simulink model "vanderpol"  (R2016a)
settings: Solver=FixedStepAuto  StartTime=0.0  StopTime=25  FixedStep=0.01  RelTol=1e-3
settings Model: Creator=kreitzem  LastModifiedBy=kreitzem

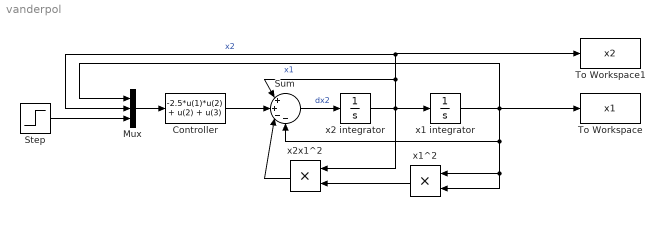
== system vanderpol ==
  Controller : Fcn  Expr=-2.5*u(1)*u(2) + u(2) + u(3)
  Mux : Mux  Inputs=3
  Step : Step  After=pi/2  SampleTime=0
  Sum : Sum  Inputs=|++--
  To Workspace : ToWorkspace  VariableName=x1  SaveFormat=Timeseries  SampleTime=-1
  To Workspace1 : ToWorkspace  VariableName=x2  SaveFormat=Timeseries  SampleTime=-1
  x1 integrator : Integrator
  x1^2 : Product
  x2 integrator : Integrator
  x2x1^2 : Product
  wires:
  x2 integrator/1 -> To Workspace1/1, Mux/2, Sum/1, x2x1^2/1, x1 integrator/1  "x2"
  Sum/1 -> x2 integrator/1  "dx2"
  x1 integrator/1 -> Mux/1, To Workspace/1, x1^2/2, x1^2/1, Sum/4  "x1"
  x1^2/1 -> x2x1^2/2
  x2x1^2/1 -> Sum/3
  Controller/1 -> Sum/2
  Mux/1 -> Controller/1
  Step/1 -> Mux/3
